simulink model "test_dram_vacc_out"  (Simulink 6.2)
settings: Solver=ode45  StartTime=0.0  StopTime=30000  RelTol=1e-3
undefined symbols (not defined in the file): ant_bits, blockCountBits, blockRowBits
libraries: xbsIndex_r3 x678, xps_library x31, casper_library x10
(part 3 of 4)

== system test_dram_vacc_out/dram_vacc1/test_address ==
  address : Inport  Port=1  LatchInput=off
  RWn : Inport  Port=2  LatchInput=off
  cmd_valid : Inport  Port=3  LatchInput=off
  Concat : xbsIndex_r3/Concat  num_inputs=3  explicit_period=on  period=1  dbl_ovrd=off
  Counter : xbsIndex_r3/Counter  cnt_type=Count Limited  n_bits=11  bin_pt=0  arith_type=Unsigned  start_count=0  cnt_to=Inf  cnt_by_val=1  operation=Up  explicit_period=off  period=1  load_pin=off  rst=off  en=on  dbl_ovrd=off  show_param=off  use_rpm=on  gen_core=off
      settings: xl_area=[0, 0, 0, 0, 0, 0, 0]
  Gateway Out1 : xbsIndex_r3/Gateway Out  output_type=Double  nbits=8  bin_pt=6  arith_type=Boolean  quantization=Truncate  overflow=Wrap  hdl_port=off  timing_constraint=None  locs_specified=off  LOCs={}  needs_fixed_name=off  show_param=off
      settings: xl_area=[0, 0, 0, 0, 0, 0, 0]
  Gateway Out39 : xbsIndex_r3/Gateway Out  output_type=Double  nbits=8  bin_pt=6  arith_type=Boolean  quantization=Truncate  overflow=Wrap  hdl_port=off  timing_constraint=None  locs_specified=off  LOCs={}  needs_fixed_name=off  show_param=off
      settings: xl_area=[0, 0, 0, 0, 0, 0, 0]
  Gateway Out43 : xbsIndex_r3/Gateway Out  output_type=Double  nbits=8  bin_pt=6  arith_type=Boolean  quantization=Truncate  overflow=Wrap  hdl_port=off  timing_constraint=None  locs_specified=off  LOCs={}  needs_fixed_name=off  show_param=off
      settings: xl_area=[0, 0, 0, 0, 0, 0, 0]
  Inverter2 : xbsIndex_r3/Inverter  latency=0  explicit_period=off  period=1  en=off  dbl_ovrd=off  show_param=off
      settings: xl_area=[0, 0, 0, 0, 0, 0, 0]
  Logical2 : xbsIndex_r3/Logical  logical_function=AND  inputs=2  precision=Full  arith_type=Unsigned  n_bits=8  bin_pt=2  align_bp=on  latency=0  explicit_period=off  period=1  en=off  dbl_ovrd=off  show_param=off
      settings: xl_area=[0, 0, 0, 0, 0, 0, 0]
  Register : xbsIndex_r3/Register  init=0  reg_only_valid=off  explicit_period=off  period=1  rst=off  en=on  out_en=off  dbl_ovrd=off  show_param=off
      settings: xl_area=[0, 0, 0, 0, 0, 0, 0]
  Register1 : xbsIndex_r3/Register  init=0  reg_only_valid=off  explicit_period=off  period=1  rst=off  en=off  out_en=off  dbl_ovrd=off  show_param=off
      settings: xl_area=[0, 0, 0, 0, 0, 0, 0]
  Relational : xbsIndex_r3/Relational  mode=a!=b  latency=1  explicit_period=off  period=1  en=on  dbl_ovrd=off  show_param=off
      settings: xl_area=[0, 0, 0, 0, 0, 0, 0]
  Scope2 : Scope  NumInputPorts=3
      settings: YMin=8.55~0.95~-1  YMax=9.45~1.05~1  SaveName=ScopeData10
  Slice1 : xbsIndex_r3/Slice  mode=Lower Bit Location + Width  nbits=2  bit1=0  base1=MSB of Input  bit0=28  base0=LSB of Input  boolean_output=off  explicit_period=off  period=1  dbl_ovrd=off
  Slice2 : xbsIndex_r3/Slice  mode=Lower Bit Location + Width  nbits=8  bit1=0  base1=MSB of Input  bit0=20  base0=LSB of Input  boolean_output=off  explicit_period=off  period=1  dbl_ovrd=off
  Slice3 : xbsIndex_r3/Slice  mode=Lower Bit Location + Width  nbits=1  bit1=0  base1=MSB of Input  bit0=13  base0=LSB of Input  boolean_output=off  explicit_period=off  period=1  dbl_ovrd=off
  bram : xps_library/Shared BRAM  Tag=xps:bram  arith_type="Signed  (2's comp)"  addr_width=11  data_width=32  data_bin_pt=0  init_vals=[1:2^11]  sample_rate=1
  posedge : casper_library/Misc/posedge  Tag=Rising Edge Detector
  wires:
  address/1 -> Slice1/1, Slice2/1, Slice3/1
  Slice3/1 -> Concat/1
  Slice2/1 -> Concat/2
  Slice1/1 -> Concat/3
  RWn/1 -> Inverter2/1
  cmd_valid/1 -> Logical2/2
  Inverter2/1 -> Logical2/1
  Concat/1 -> Register/1, Relational/2
  Logical2/1 -> Register/2, Relational/3
  Register/1 -> Relational/1, Register1/1
  Relational/1 -> posedge/1
  Counter/1 -> bram/1, Gateway Out39/1
  Register1/1 -> bram/2, Gateway Out43/1
  Gateway Out39/1 -> Scope2/1
  Gateway Out43/1 -> Scope2/2
  posedge/1 -> Counter/1, bram/3, Gateway Out1/1
  Gateway Out1/1 -> Scope2/3

== system test_dram_vacc_out/dram_vacc1/test_index ==
  address : Inport  Port=1  LatchInput=off
  RWn : Inport  Port=2  LatchInput=off
  cmd_valid : Inport  Port=3  LatchInput=off
  data : Inport  Port=4  LatchInput=off
  Concat1 : xbsIndex_r3/Concat  num_inputs=2  explicit_period=on  period=1  dbl_ovrd=off
  Convert : xbsIndex_r3/Convert  Orientation=up  arith_type=Boolean  n_bits=8  bin_pt=6  quantization=Truncate  overflow=Wrap  latency=0  explicit_period=on  period=1  dbl_ovrd=off  show_param=off  inserted_by_tool=off  pipeline=off
      settings: xl_area=[0, 0, 0, 0, 0, 0, 0]
  Convert1 : xbsIndex_r3/Convert  arith_type=Unsigned  n_bits=32  bin_pt=0  quantization=Truncate  overflow=Wrap  latency=0  explicit_period=on  period=1  dbl_ovrd=off  show_param=off  inserted_by_tool=off  pipeline=off
      settings: xl_area=[0, 0, 0, 0, 0, 0, 0]
  Counter : xbsIndex_r3/Counter  cnt_type=Count Limited  n_bits=13  bin_pt=0  arith_type=Unsigned  start_count=0  cnt_to=Inf  cnt_by_val=1  operation=Up  explicit_period=off  period=1  load_pin=off  rst=off  en=on  dbl_ovrd=off  show_param=off  use_rpm=on  gen_core=off
      settings: xl_area=[0, 0, 0, 0, 0, 0, 0]
  Gateway Out{1..3,39,43} (5 alike) : xbsIndex_r3/Gateway Out  output_type=Double  nbits=8  bin_pt=6  arith_type=Boolean  quantization=Truncate  overflow=Wrap  hdl_port=off  timing_constraint=None  locs_specified=off  LOCs={}  needs_fixed_name=off  show_param=off
      settings: xl_area=[0, 0, 0, 0, 0, 0, 0]
  Inverter2 : xbsIndex_r3/Inverter  latency=0  explicit_period=off  period=1  en=off  dbl_ovrd=off  show_param=off
      settings: xl_area=[0, 0, 0, 0, 0, 0, 0]
  Logical2 : xbsIndex_r3/Logical  logical_function=AND  inputs=2  precision=Full  arith_type=Unsigned  n_bits=8  bin_pt=2  align_bp=on  latency=0  explicit_period=off  period=1  en=off  dbl_ovrd=off  show_param=off
      settings: xl_area=[0, 0, 0, 0, 0, 0, 0]
  Register : xbsIndex_r3/Register  init=0  reg_only_valid=off  explicit_period=off  period=1  rst=off  en=off  out_en=off  dbl_ovrd=off  show_param=off
      settings: xl_area=[0, 0, 0, 0, 0, 0, 0]
  Relational1 : xbsIndex_r3/Relational  mode=a=b  latency=1  explicit_period=off  period=1  en=on  dbl_ovrd=off  show_param=off
      settings: xl_area=[0, 0, 0, 0, 0, 0, 0]
  Scope2 : Scope  NumInputPorts=5
      settings: YMin=13~0~0~0~0  YMax=16~1000~1~400~1  SaveName=ScopeData10
  Slice1 : xbsIndex_r3/Slice  mode=Lower Bit Location + Width  nbits=14  bit1=0  base1=MSB of Input  bit0=0  base0=LSB of Input  boolean_output=off  explicit_period=off  period=1  dbl_ovrd=off
  Slice4 : xbsIndex_r3/Slice  mode=Lower Bit Location + Width  nbits=32  bit1=0  base1=MSB of Input  bit0=0  base0=LSB of Input  boolean_output=off  explicit_period=off  period=1  dbl_ovrd=off
  bram : xps_library/Shared BRAM  Tag=xps:bram  arith_type=Unsigned  addr_width=13  data_width=32  data_bin_pt=0  init_vals=[1:2^11]  sample_rate=1
  clm_slice : xbsIndex_r3/Slice  mode=Lower Bit Location + Width  nbits=8  bit1=0  base1=MSB of Input  bit0=5  base0=LSB of Input  boolean_output=off  explicit_period=off  period=1  dbl_ovrd=off
  cnt : xps_library/software register  Tag=xps:sw_reg  io_dir=To Processor  arith_type=Unsigned  bitwidth=32  bin_pt=0  sample_period=1  gw_name=test_dram_vacc_out_dram_vacc1_test_index_cnt_user_data_in
  master_reset_sim1 : Constant  Value=4
  posedge2 : casper_library/Misc/posedge  Tag=Rising Edge Detector
  position : xps_library/software register  Tag=xps:sw_reg  io_dir=From Processor  arith_type=Unsigned  bitwidth=32  bin_pt=0  sample_period=1  gw_name=test_dram_vacc_out_dram_vacc1_test_index_position_user_data_out
  row_slice : xbsIndex_r3/Slice  mode=Lower Bit Location + Width  nbits=6  bit1=0  base1=MSB of Input  bit0=14  base0=LSB of Input  boolean_output=off  explicit_period=off  period=1  dbl_ovrd=off
  wires:
  Gateway Out43/1 -> Scope2/2
  Gateway Out39/1 -> Scope2/1
  Counter/1 -> bram/1, Gateway Out39/1, Convert1/1
  Inverter2/1 -> Logical2/1
  cmd_valid/1 -> Logical2/2
  RWn/1 -> Inverter2/1
  address/1 -> clm_slice/1, row_slice/1
  master_reset_sim1/1 -> position/1
  data/1 -> Slice4/1
  row_slice/1 -> Concat1/1
  clm_slice/1 -> Concat1/2
  position/1 -> Slice1/1
  Concat1/1 -> Relational1/2, Gateway Out2/1
  Logical2/1 -> Convert/1, Gateway Out3/1
  Relational1/1 -> posedge2/1
  posedge2/1 -> Counter/1, bram/3, Gateway Out1/1
  Slice4/1 -> Register/1
  Gateway Out1/1 -> Scope2/3
  Register/1 -> bram/2, Gateway Out43/1
  Slice1/1 -> Relational1/1
  Convert/1 -> Relational1/3
  Convert1/1 -> cnt/1
  Gateway Out2/1 -> Scope2/4
  Gateway Out3/1 -> Scope2/5

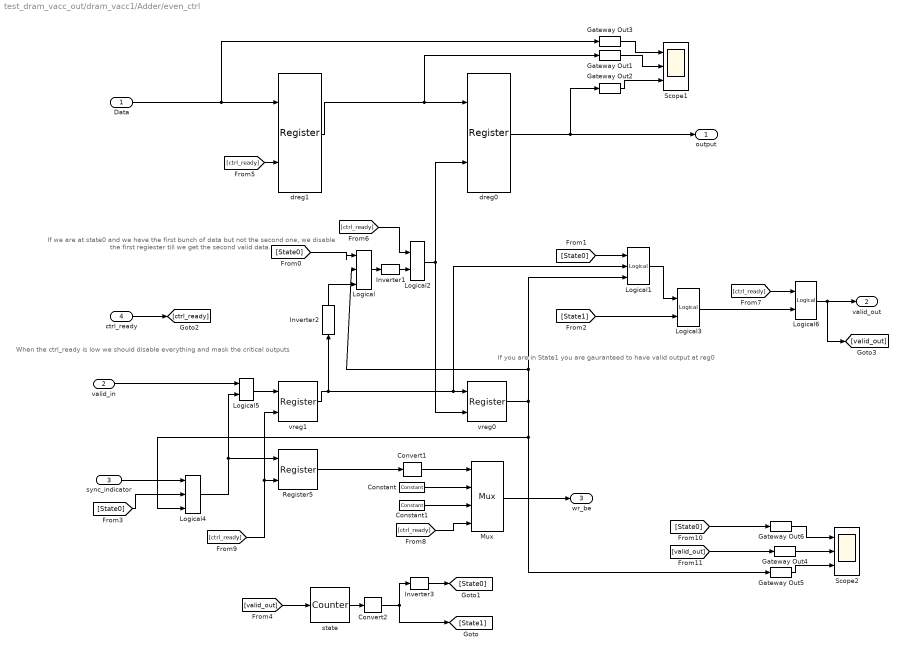
== system test_dram_vacc_out/dram_vacc1/Adder/even_ctrl ==
  note: If we are at state0
      | and we have the first bunch of data
      | but not the second one,
      | we disable the first regiester till we
      | get the second valid  data.
  note: When the ctrl_ready is low
      | we should disable everything
      | and mask the critical outputs
  note: If you are in State1
      | you are gauranteed to have
      | valid output at reg0
  Data : Inport  Port=1  LatchInput=off
  valid_in : Inport  Port=2  LatchInput=off
  sync_indicator : Inport  Port=3  LatchInput=off
  ctrl_ready : Inport  Port=4  LatchInput=off
  Constant : xbsIndex_r3/Constant  const=2^18-1  equ=P=C  arith_type=Unsigned  n_bits=18  bin_pt=0  opselect=C  inp2=PCIN>>17  opr=+  inp1=P  carry=CIN  iostate=0  explicit_period=on  period=1  dbl_ovrd=off
  Constant1 : xbsIndex_r3/Constant  const=0  equ=P=C  arith_type=Unsigned  n_bits=18  bin_pt=0  opselect=C  inp2=PCIN>>17  opr=+  inp1=P  carry=CIN  iostate=0  explicit_period=on  period=1  dbl_ovrd=off
  Convert1 : xbsIndex_r3/Convert  arith_type=Boolean  n_bits=1  bin_pt=0  quantization=Truncate  overflow=Wrap  latency=0  explicit_period=off  period=1  dbl_ovrd=off  show_param=off  inserted_by_tool=off  pipeline=off
      settings: xl_area=[0, 0, 0, 0, 0, 0, 0]
  Convert2 : xbsIndex_r3/Convert  arith_type=Boolean  n_bits=1  bin_pt=0  quantization=Truncate  overflow=Wrap  latency=0  explicit_period=off  period=1  dbl_ovrd=off  show_param=off  inserted_by_tool=off  pipeline=off
      settings: xl_area=[0, 0, 0, 0, 0, 0, 0]
  Gateway Out{1..6} (6 alike) : xbsIndex_r3/Gateway Out  output_type=Double  nbits=8  bin_pt=6  arith_type=Boolean  quantization=Truncate  overflow=Wrap  hdl_port=off  timing_constraint=None  locs_specified=off  LOCs={}  needs_fixed_name=off  show_param=off
      settings: xl_area=[0, 0, 0, 0, 0, 0, 0]
  Inverter1 : xbsIndex_r3/Inverter  latency=0  explicit_period=off  period=1  en=off  dbl_ovrd=off  show_param=off
      settings: xl_area=[0, 0, 0, 0, 0, 0, 0]
  Inverter2 : xbsIndex_r3/Inverter  Orientation=up  latency=0  explicit_period=off  period=1  en=off  dbl_ovrd=off  show_param=off
      settings: xl_area=[0, 0, 0, 0, 0, 0, 0]
  Inverter3 : xbsIndex_r3/Inverter  latency=0  explicit_period=off  period=1  en=off  dbl_ovrd=off  show_param=off
      settings: xl_area=[0, 0, 0, 0, 0, 0, 0]
  Logical : xbsIndex_r3/Logical  logical_function=AND  inputs=3  precision=Full  arith_type=Unsigned  n_bits=8  bin_pt=2  align_bp=on  latency=0  explicit_period=off  period=1  en=off  dbl_ovrd=off  show_param=off
      settings: xl_area=[0, 0, 0, 0, 0, 0, 0]
  Logical1 : xbsIndex_r3/Logical  logical_function=AND  inputs=3  precision=Full  arith_type=Unsigned  n_bits=8  bin_pt=2  align_bp=on  latency=0  explicit_period=off  period=1  en=off  dbl_ovrd=off  show_param=off
      settings: xl_area=[0, 0, 0, 0, 0, 0, 0]
  Logical2 : xbsIndex_r3/Logical  logical_function=AND  inputs=2  precision=Full  arith_type=Unsigned  n_bits=8  bin_pt=2  align_bp=on  latency=0  explicit_period=off  period=1  en=off  dbl_ovrd=off  show_param=off
      settings: xl_area=[0, 0, 0, 0, 0, 0, 0]
  Logical3 : xbsIndex_r3/Logical  logical_function=OR  inputs=2  precision=Full  arith_type=Unsigned  n_bits=8  bin_pt=2  align_bp=on  latency=0  explicit_period=off  period=1  en=off  dbl_ovrd=off  show_param=off
      settings: xl_area=[0, 0, 0, 0, 0, 0, 0]
  Logical4 : xbsIndex_r3/Logical  logical_function=AND  inputs=3  precision=Full  arith_type=Unsigned  n_bits=8  bin_pt=2  align_bp=on  latency=0  explicit_period=off  period=1  en=off  dbl_ovrd=off  show_param=off
      settings: xl_area=[0, 0, 0, 0, 0, 0, 0]
  Logical5 : xbsIndex_r3/Logical  logical_function=OR  inputs=2  precision=Full  arith_type=Unsigned  n_bits=8  bin_pt=2  align_bp=on  latency=0  explicit_period=off  period=1  en=off  dbl_ovrd=off  show_param=off
      settings: xl_area=[0, 0, 0, 0, 0, 0, 0]
  Logical6 : xbsIndex_r3/Logical  logical_function=AND  inputs=2  precision=Full  arith_type=Unsigned  n_bits=8  bin_pt=2  align_bp=on  latency=0  explicit_period=off  period=1  en=off  dbl_ovrd=off  show_param=off
      settings: xl_area=[0, 0, 0, 0, 0, 0, 0]
  Mux : xbsIndex_r3/Mux  inputs=2  precision=Full  arith_type="Signed  (2's comp)"  n_bits=8  bin_pt=2  quantization=Truncate  overflow=Wrap  latency=1  explicit_period=off  period=1  en=on  dbl_ovrd=off  show_param=off  mux_type=off  use_rpm=off  gen_core=off
      settings: xl_area=[0, 0, 0, 0, 0, 0, 0]
  Register5 : xbsIndex_r3/Register  init=0  reg_only_valid=off  explicit_period=off  period=1  rst=off  en=on  out_en=off  dbl_ovrd=off  show_param=off
      settings: xl_area=[0, 0, 0, 0, 0, 0, 0]
  Scope1 : Scope  NumInputPorts=3
      settings: YMin=0~0~0  YMax=1100~1~1  SaveName=ScopeData2
  Scope2 : Scope  NumInputPorts=3
      settings: YMin=0~0~0  YMax=1100~1~1
  dreg0 : xbsIndex_r3/Register  init=0  reg_only_valid=off  explicit_period=on  period=1  rst=off  en=on  out_en=off  dbl_ovrd=off  show_param=off
      settings: xl_area=[0, 0, 0, 0, 0, 0, 0]
  dreg1 : xbsIndex_r3/Register  init=0  reg_only_valid=off  explicit_period=off  period=1  rst=off  en=on  out_en=off  dbl_ovrd=off  show_param=off
      settings: xl_area=[0, 0, 0, 0, 0, 0, 0]
  state : xbsIndex_r3/Counter  cnt_type=Free Running  n_bits=1  bin_pt=0  arith_type=Unsigned  start_count=0  cnt_to=Inf  cnt_by_val=1  operation=Up  explicit_period=on  period=1  load_pin=off  rst=off  en=on  dbl_ovrd=off  show_param=off  use_rpm=on  gen_core=off
      settings: xl_area=[0, 0, 0, 0, 0, 0, 0]
  vreg0 : xbsIndex_r3/Register  init=0  reg_only_valid=off  explicit_period=on  period=1  rst=off  en=on  out_en=off  dbl_ovrd=off  show_param=off
      settings: xl_area=[0, 0, 0, 0, 0, 0, 0]
  vreg1 : xbsIndex_r3/Register  init=0  reg_only_valid=off  explicit_period=on  period=1  rst=off  en=on  out_en=off  dbl_ovrd=off  show_param=off
      settings: xl_area=[0, 0, 0, 0, 0, 0, 0]
  output : Outport
  valid_out : Outport  Port=2
  wr_be : Outport  Port=3
  wires:
  Data/1 -> dreg1/1, Gateway Out3/1
  valid_in/1 -> Logical5/1
  vreg1/1 -> vreg0/1, Logical1/2, Inverter2/1
  dreg1/1 -> dreg0/1, Gateway Out1/1
  dreg0/1 -> output/1, Gateway Out2/1
  state/1 -> Convert2/1
  [State0] -> Logical/1
  vreg0/1 -> Logical/2, Logical1/3, Logical4/3, Gateway Out5/1
  Logical/1 -> Inverter1/1
  [State0] -> Logical1/1
  Inverter3/1 -> [State0]
  [State1] -> Logical3/2
  Logical1/1 -> Logical3/1
  ctrl_ready/1 -> [ctrl_ready]
  Logical3/1 -> Logical6/2
  Inverter2/1 -> Logical/3
  [valid_out] -> state/1
  sync_indicator/1 -> Logical4/1
  [State0] -> Logical4/2
  Mux/1 -> wr_be/1
  Logical5/1 -> vreg1/1
  Logical4/1 -> Logical5/2, Register5/1
  Register5/1 -> Convert1/1
  Constant/1 -> Mux/2
  Constant1/1 -> Mux/3
  [ctrl_ready] -> dreg1/2
  Logical6/1 -> valid_out/1, [valid_out]
  [ctrl_ready] -> Logical6/1
  [ctrl_ready] -> Mux/4
  [ctrl_ready] -> vreg1/2, Register5/2
  Gateway Out6/1 -> Scope2/1
  Gateway Out4/1 -> Scope2/2
  Gateway Out5/1 -> Scope2/3
  [State0] -> Gateway Out6/1
  [valid_out] -> Gateway Out4/1
  Gateway Out3/1 -> Scope1/1
  Gateway Out1/1 -> Scope1/2
  Gateway Out2/1 -> Scope1/3
  Convert1/1 -> Mux/1
  Convert2/1 -> [State1], Inverter3/1
  Inverter1/1 -> Logical2/2
  [ctrl_ready] -> Logical2/1
  Logical2/1 -> dreg0/2, vreg0/2

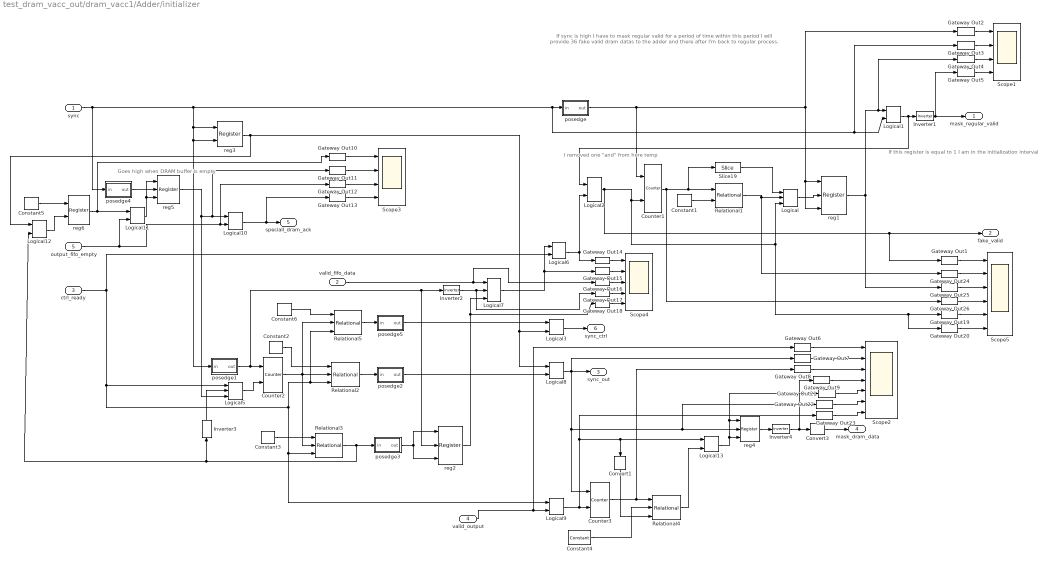
== system test_dram_vacc_out/dram_vacc1/Adder/initializer ==
  note: I removed one "and"
      | from here temp
  note: If this register is equal to 1 I am
      | in the initialization interval
  note: If sync is high I have to mask regular valid for a period of time
      | within this period I will provide 36 fake valid dram datas to the adder and there after I'm back to
      | regular process.
  note: Goes high when DRAM
      | buffer is empty
  sync : Inport  Port=1  LatchInput=off
  valid_fifo_data : Inport  Port=2  LatchInput=off
  ctrl_ready : Inport  Port=3  LatchInput=off
  valid_output : Inport  Port=4  LatchInput=off
  output_fifo_empty : Inport  Port=5  LatchInput=off
  Constant1 : xbsIndex_r3/Constant  const=34  equ=P=C  arith_type=Unsigned  n_bits=6  bin_pt=0  opselect=C  inp2=PCIN>>17  opr=+  inp1=P  carry=CIN  iostate=0  explicit_period=on  period=1  dbl_ovrd=off
  Constant2 : xbsIndex_r3/Constant  const=7  equ=P=C  arith_type=Unsigned  n_bits=4  bin_pt=0  opselect=C  inp2=PCIN>>17  opr=+  inp1=P  carry=CIN  iostate=0  explicit_period=on  period=1  dbl_ovrd=off
  Constant3 : xbsIndex_r3/Constant  const=14  equ=P=C  arith_type=Unsigned  n_bits=4  bin_pt=0  opselect=C  inp2=PCIN>>17  opr=+  inp1=P  carry=CIN  iostate=0  explicit_period=on  period=1  dbl_ovrd=off
  Constant4 : xbsIndex_r3/Constant  const=acc_length-2  equ=P=C  arith_type=Unsigned  n_bits=22  bin_pt=0  opselect=C  inp2=PCIN>>17  opr=+  inp1=P  carry=CIN  iostate=0  explicit_period=on  period=1  dbl_ovrd=off
  Constant5 : xbsIndex_r3/Constant  const=0  equ=P=C  arith_type=Boolean  n_bits=4  bin_pt=0  opselect=C  inp2=PCIN>>17  opr=+  inp1=P  carry=CIN  iostate=0  explicit_period=on  period=1  dbl_ovrd=off
  Constant6 : xbsIndex_r3/Constant  const=4  equ=P=C  arith_type=Unsigned  n_bits=4  bin_pt=0  opselect=C  inp2=PCIN>>17  opr=+  inp1=P  carry=CIN  iostate=0  explicit_period=on  period=1  dbl_ovrd=off
  Convert1 : xbsIndex_r3/Convert  Orientation=down  arith_type=Boolean  n_bits=1  bin_pt=0  quantization=Truncate  overflow=Wrap  latency=0  explicit_period=off  period=1  dbl_ovrd=off  show_param=off  inserted_by_tool=off  pipeline=off
      settings: xl_area=[0, 0, 0, 0, 0, 0, 0]
  Convert3 : xbsIndex_r3/Convert  arith_type=Unsigned  n_bits=1  bin_pt=0  quantization=Truncate  overflow=Wrap  latency=0  explicit_period=off  period=1  dbl_ovrd=off  show_param=off  inserted_by_tool=off  pipeline=off
      settings: xl_area=[0, 0, 0, 0, 0, 0, 0]
  Counter1 : xbsIndex_r3/Counter  cnt_type=Count Limited  n_bits=6  bin_pt=0  arith_type=Unsigned  start_count=0  cnt_to=35  cnt_by_val=1  operation=Up  explicit_period=on  period=1  load_pin=off  rst=on  en=on  dbl_ovrd=off  show_param=off  use_rpm=on  gen_core=off
      settings: xl_area=[0, 0, 0, 0, 0, 0, 0]
  Counter2 : xbsIndex_r3/Counter  cnt_type=Free Running  n_bits=4  bin_pt=0  arith_type=Unsigned  start_count=0  cnt_to=35  cnt_by_val=1  operation=Up  explicit_period=on  period=1  load_pin=off  rst=on  en=on  dbl_ovrd=off  show_param=off  use_rpm=on  gen_core=off
      settings: xl_area=[0, 0, 0, 0, 0, 0, 0]
  Counter3 : xbsIndex_r3/Counter  cnt_type=Free Running  n_bits=22  bin_pt=0  arith_type=Unsigned  start_count=0  cnt_to=35  cnt_by_val=1  operation=Up  explicit_period=on  period=1  load_pin=off  rst=on  en=on  dbl_ovrd=off  show_param=off  use_rpm=on  gen_core=off
      settings: xl_area=[0, 0, 0, 0, 0, 0, 0]
  Gateway Out{1..26} (26 alike) : xbsIndex_r3/Gateway Out  output_type=Double  nbits=8  bin_pt=6  arith_type=Boolean  quantization=Truncate  overflow=Wrap  hdl_port=off  timing_constraint=None  locs_specified=off  LOCs={}  needs_fixed_name=off  show_param=off
      settings: xl_area=[0, 0, 0, 0, 0, 0, 0]
  Inverter1 : xbsIndex_r3/Inverter  latency=0  explicit_period=off  period=1  en=off  dbl_ovrd=off  show_param=off
      settings: xl_area=[0, 0, 0, 0, 0, 0, 0]
  Inverter2 : xbsIndex_r3/Inverter  latency=0  explicit_period=off  period=1  en=off  dbl_ovrd=off  show_param=off
      settings: xl_area=[0, 0, 0, 0, 0, 0, 0]
  Inverter3 : xbsIndex_r3/Inverter  Orientation=up  latency=0  explicit_period=off  period=1  en=off  dbl_ovrd=off  show_param=off
      settings: xl_area=[0, 0, 0, 0, 0, 0, 0]
  Inverter4 : xbsIndex_r3/Inverter  latency=0  explicit_period=off  period=1  en=off  dbl_ovrd=off  show_param=off
      settings: xl_area=[0, 0, 0, 0, 0, 0, 0]
  Logical : xbsIndex_r3/Logical  logical_function=AND  inputs=3  precision=Full  arith_type=Unsigned  n_bits=8  bin_pt=2  align_bp=on  latency=0  explicit_period=on  period=1  en=off  dbl_ovrd=off  show_param=off
      settings: xl_area=[0, 0, 0, 0, 0, 0, 0]
  Logical1 : xbsIndex_r3/Logical  logical_function=OR  inputs=2  precision=Full  arith_type=Unsigned  n_bits=8  bin_pt=2  align_bp=on  latency=0  explicit_period=off  period=1  en=off  dbl_ovrd=off  show_param=off
      settings: xl_area=[0, 0, 0, 0, 0, 0, 0]
  Logical10 : xbsIndex_r3/Logical  logical_function=NOR  inputs=2  precision=Full  arith_type=Unsigned  n_bits=8  bin_pt=2  align_bp=on  latency=0  explicit_period=off  period=1  en=off  dbl_ovrd=off  show_param=off
      settings: xl_area=[0, 0, 0, 0, 0, 0, 0]
  Logical11 : xbsIndex_r3/Logical  logical_function=OR  inputs=2  precision=Full  arith_type=Unsigned  n_bits=8  bin_pt=2  align_bp=on  latency=0  explicit_period=off  period=1  en=off  dbl_ovrd=off  show_param=off
      settings: xl_area=[0, 0, 0, 0, 0, 0, 0]
  Logical{2..3,6,8..9,12..13} (7 alike) : xbsIndex_r3/Logical  logical_function=AND  inputs=2  precision=Full  arith_type=Unsigned  n_bits=8  bin_pt=2  align_bp=on  latency=0  explicit_period=off  period=1  en=off  dbl_ovrd=off  show_param=off
      settings: xl_area=[0, 0, 0, 0, 0, 0, 0]
  Logical5 : xbsIndex_r3/Logical  logical_function=AND  inputs=3  precision=Full  arith_type=Unsigned  n_bits=8  bin_pt=2  align_bp=on  latency=0  explicit_period=off  period=1  en=off  dbl_ovrd=off  show_param=off
      settings: xl_area=[0, 0, 0, 0, 0, 0, 0]
  Logical7 : xbsIndex_r3/Logical  logical_function=AND  inputs=3  precision=Full  arith_type=Unsigned  n_bits=8  bin_pt=2  align_bp=on  latency=0  explicit_period=off  period=1  en=off  dbl_ovrd=off  show_param=off
      settings: xl_area=[0, 0, 0, 0, 0, 0, 0]
  Relational1 : xbsIndex_r3/Relational  mode=a>=b  latency=1  explicit_period=on  period=1  en=off  dbl_ovrd=off  show_param=off
      settings: xl_area=[0, 0, 0, 0, 0, 0, 0]
  Relational2 : xbsIndex_r3/Relational  mode=a<=b  latency=1  explicit_period=on  period=1  en=on  dbl_ovrd=off  show_param=off
      settings: xl_area=[0, 0, 0, 0, 0, 0, 0]
  Relational3 : xbsIndex_r3/Relational  mode=a<=b  latency=1  explicit_period=on  period=1  en=on  dbl_ovrd=off  show_param=off
      settings: xl_area=[0, 0, 0, 0, 0, 0, 0]
  Relational4 : xbsIndex_r3/Relational  mode=a=b  latency=1  explicit_period=on  period=1  en=on  dbl_ovrd=off  show_param=off
      settings: xl_area=[0, 0, 0, 0, 0, 0, 0]
  Relational5 : xbsIndex_r3/Relational  mode=a<=b  latency=1  explicit_period=on  period=1  en=on  dbl_ovrd=off  show_param=off
      settings: xl_area=[0, 0, 0, 0, 0, 0, 0]
  Scope1 : Scope  NumInputPorts=4
      settings: YMin=-1~-1~50~0  YMax=1~1~90~1  SaveName=ScopeData13
  Scope2 : Scope  NumInputPorts=7
      settings: YMin=-1~-1~50~0~-5~-5~-5  YMax=1~1~90~1~5~5~5  SaveName=ScopeData15
  Scope3 : Scope  NumInputPorts=4
      settings: YMin=-1~-1~50~0  YMax=1~1~90~1  SaveName=ScopeData18
  Scope4 : Scope  NumInputPorts=5
      settings: YMin=-1~-1~50~0~-5  YMax=1~1~90~1~5  SaveName=ScopeData31
  Scope5 : Scope  NumInputPorts=6
      settings: YMin=-1~-1~50~0~-5~-5  YMax=1~1~90~1~5~5  SaveName=ScopeData3
  Slice19 : xbsIndex_r3/Slice  mode=Lower Bit Location + Width  nbits=1  bit1=0  base1=MSB of Input  bit0=0  base0=LSB of Input  boolean_output=on  explicit_period=off  period=1  dbl_ovrd=off
  posedge : Subsystem
  posedge1 : Subsystem
  posedge2 : Subsystem
  posedge3 : Subsystem
  posedge4 : Subsystem
  posedge5 : Subsystem
  reg{1..2,4..5} (4 alike) : xbsIndex_r3/Register  init=0  reg_only_valid=off  explicit_period=on  period=1  rst=on  en=on  out_en=off  dbl_ovrd=off  show_param=off
      settings: xl_area=[0, 0, 0, 0, 0, 0, 0]
  reg3 : xbsIndex_r3/Register  init=0  reg_only_valid=off  explicit_period=on  period=1  rst=off  en=on  out_en=off  dbl_ovrd=off  show_param=off
      settings: xl_area=[0, 0, 0, 0, 0, 0, 0]
  reg6 : xbsIndex_r3/Register  init=1  reg_only_valid=off  explicit_period=on  period=1  rst=off  en=on  out_en=off  dbl_ovrd=off  show_param=off
      settings: xl_area=[0, 0, 0, 0, 0, 0, 0]
  mask_regular_valid : Outport
  fake_valid : Outport  Port=2
  sync_out : Outport  Port=3
  mask_dram_data : Outport  Port=4
  speciall_dram_ack : Outport  Port=5
  sync_ctrl : Outport  Port=6
  wires:
  Convert1/1 -> Relational4/3
  Gateway Out23/1 -> Scope2/7
  Gateway Out22/1 -> Scope2/6
  Gateway Out21/1 -> Scope2/5
  Slice19/1 -> Logical/1
  Gateway Out20/1 -> Scope5/6
  Gateway Out19/1 -> Scope5/5
  Gateway Out18/1 -> Scope4/5
  Gateway Out17/1 -> Scope4/4
  Gateway Out16/1 -> Scope4/3
  Gateway Out15/1 -> Scope4/2
  Gateway Out14/1 -> Scope4/1
  Convert3/1 -> mask_dram_data/1
  Relational4/1 -> Logical13/2
  Logical13/1 -> Gateway Out21/1, reg4/1, reg4/3
  reg6/1 -> Gateway Out10/1, Logical11/1
  Logical12/1 -> reg6/2
  Constant5/1 -> reg6/1
  Gateway Out10/1 -> Scope3/1
  Gateway Out13/1 -> Scope3/4
  Gateway Out12/1 -> Scope3/3
  Gateway Out11/1 -> Scope3/2
  Logical11/1 -> reg5/3, reg5/1
  Logical10/1 -> Gateway Out13/1, speciall_dram_ack/1
  output_fifo_empty/1 -> Gateway Out12/1, Logical10/2, Logical11/2
  reg5/1 -> Gateway Out11/1, Logical10/1, Logical5/3
  posedge4/1(out) -> reg5/2
  Gateway Out6/1 -> Scope2/1
  Gateway Out9/1 -> Scope2/4
  Gateway Out8/1 -> Scope2/3
  Gateway Out7/1 -> Scope2/2
  Inverter4/1 -> Convert3/1, Gateway Out9/1
  reg4/1 -> Inverter4/1
  Constant4/1 -> Relational4/2
  Counter3/1 -> Gateway Out8/1, Relational4/1
  valid_output/1 -> Gateway Out6/1, Logical9/2
  Logical9/1 -> Convert1/1, Logical13/1, Gateway Out23/1, Counter3/2
  reg3/1 -> Logical12/1, Logical8/1, Logical3/2
  posedge2/1(out) -> Logical8/2
  Logical8/1 -> Gateway Out7/1, Gateway Out22/1, reg4/2, Counter3/1, sync_out/1
  Inverter3/1 -> Logical5/2
  Logical5/1 -> Counter2/2
  Logical7/1 -> Gateway Out15/1, Logical6/1
  valid_fifo_data/1 -> Gateway Out16/1, Logical7/1
  Inverter2/1 -> Gateway Out17/1, Logical7/2
  reg2/1 -> Gateway Out18/1, Logical7/3
  posedge3/1(out) -> reg2/3, reg2/1
  Relational3/1 -> Logical12/2, Inverter3/1, posedge3/1(in)
  Constant3/1 -> Relational3/1
  Relational2/1 -> posedge2/1(in)
  Constant2/1 -> Relational2/1
  Counter2/1 -> Relational3/2, Relational2/2, Relational5/2
  posedge1/1(out) -> Inverter2/1, reg2/2, Counter2/1
  Inverter1/1 -> Gateway Out5/1, mask_regular_valid/1
  Logical/1 -> reg1/2
  Logical6/1 -> Gateway Out14/1, Logical2/2
  ctrl_ready/1 -> Logical9/1, Relational3/3, Relational2/3, Relational5/3, Logical5/1, Logical6/2
  Relational1/1 -> Logical/2, Gateway Out24/1
  reg1/1 -> Gateway Out25/1, Gateway Out4/1, Logical1/1
  Constant1/1 -> Relational1/2
  Counter1/1 -> Slice19/1, Relational1/1, Gateway Out26/1
  Logical2/1 -> Counter1/2, Gateway Out20/1, Gateway Out19/1, Logical/3, Gateway Out1/1, fake_valid/1
  Logical1/1 -> Logical2/1, Inverter1/1
  posedge/1(out) -> Counter1/1, reg1/3, reg1/1, Gateway Out2/1
  sync/1 -> posedge4/1(in), reg3/1, reg3/2, posedge1/1(in), Gateway Out3/1, Logical1/2, posedge/1(in)
  Gateway Out2/1 -> Scope1/1
  Gateway Out5/1 -> Scope1/4
  Gateway Out4/1 -> Scope1/3
  Gateway Out3/1 -> Scope1/2
  Gateway Out1/1 -> Scope5/1
  Gateway Out26/1 -> Scope5/4
  Gateway Out25/1 -> Scope5/3
  Gateway Out24/1 -> Scope5/2
  Constant6/1 -> Relational5/1
  Relational5/1 -> posedge5/1(in)
  posedge5/1(out) -> Logical3/1
  Logical3/1 -> sync_ctrl/1

== system test_dram_vacc_out/dram_vacc1/RB_reg/Trickle_FWFT ==
  note: We needed a FIFO which brings the valid data automatically to the output.
      | The regular XILINX Fifos are not FWFT (First Word Fall Through).
      | We tried to make one but it was really hard to make one agreeing with the exact specs.
      | This module which we have named it Trickle_FWFT Fifo works very similiarly with minor
      | differences which servers our purpose here in the DRAM VACC module.
  note: The real depth of this module is depth+1.
      | The valid signal will go high with one cycle delay.
  din : Inport  Port=1  LatchInput=off
  we : Inport  Port=2  LatchInput=off
  ack : Inport  Port=3  LatchInput=off
  reset : Inport  Port=4  LatchInput=off
  Convert : xbsIndex_r3/Convert  Orientation=left  arith_type=Boolean  n_bits=8  bin_pt=6  quantization=Truncate  overflow=Wrap  latency=0  explicit_period=on  period=1  dbl_ovrd=off  show_param=off  inserted_by_tool=off  pipeline=off
      settings: xl_area=[0, 0, 0, 0, 0, 0, 0]
  Convert3 : xbsIndex_r3/Convert  arith_type=Boolean  n_bits=8  bin_pt=6  quantization=Truncate  overflow=Wrap  latency=0  explicit_period=off  period=1  dbl_ovrd=off  show_param=off  inserted_by_tool=off  pipeline=off
      settings: xl_area=[0, 0, 0, 0, 0, 0, 0]
  FIFO : xbsIndex_r3/FIFO  depth=16  percent_nbits=1  store_only_valid=on  init_zero=on  explicit_period=on  period=1  rst=on  en=off  use_almost_empty=off  almost_empty_offset=6  use_almost_full=off  almost_full_offset=6  dbl_ovrd=off  show_param=off  mem_type=Block RAM  gen_core=off
      settings: xl_area=[0, 0, 0, 0, 0, 0, 0]
  Inverter3 : xbsIndex_r3/Inverter  latency=0  explicit_period=off  period=1  en=off  dbl_ovrd=off  show_param=off
      settings: xl_area=[0, 0, 0, 0, 0, 0, 0]
  Logical2 : xbsIndex_r3/Logical  logical_function=OR  inputs=2  precision=Full  arith_type=Unsigned  n_bits=8  bin_pt=2  align_bp=on  latency=0  explicit_period=on  period=1  en=off  dbl_ovrd=off  show_param=off
      settings: xl_area=[0, 0, 0, 0, 0, 0, 0]
  not_valid : xbsIndex_r3/Register  init=1  reg_only_valid=off  explicit_period=on  period=1  rst=on  en=on  out_en=off  dbl_ovrd=off  show_param=off
      settings: xl_area=[0, 0, 0, 0, 0, 0, 0]
  data_out : Outport
  valid : Outport  Port=2
  full : Outport  Port=3
  %full : Outport  Port=4
  wires:
  din/1 -> FIFO/1
  we/1 -> FIFO/2
  FIFO/2 -> not_valid/1
  ack/1 -> Logical2/2
  FIFO/1 -> data_out/1
  FIFO/4 -> full/1
  Inverter3/1 -> Convert3/1
  reset/1 -> FIFO/4, not_valid/2
  Logical2/1 -> FIFO/3, not_valid/3
  not_valid/1 -> Inverter3/1, Convert/1
  Convert/1 -> Logical2/1
  FIFO/3 -> %full/1
  Convert3/1 -> valid/1

== system test_dram_vacc_out/dram_vacc1/RB_reg/er ==
  dout : Inport  Port=1  LatchInput=off
  valid : Inport  Port=2  LatchInput=off
  Constant : xbsIndex_r3/Constant  const=1  equ=P=C  arith_type=Unsigned  n_bits=128  bin_pt=0  opselect=C  inp2=PCIN>>17  opr=+  inp1=P  carry=CIN  iostate=0  explicit_period=on  period=1  dbl_ovrd=off
  Constant1 : Constant  Value=0
  Delay : xbsIndex_r3/Delay  latency=3  reg_retiming=off  explicit_period=off  period=1  en=off  accept_only_valid=off  init_zero=on  dbl_ovrd=off  show_param=off
      settings: xl_area=[0, 0, 0, 0, 0, 0, 0]
  Logical : xbsIndex_r3/Logical  logical_function=AND  inputs=2  precision=Full  arith_type=Unsigned  n_bits=8  bin_pt=2  align_bp=on  latency=0  explicit_period=off  period=1  en=off  dbl_ovrd=off  show_param=off
      settings: xl_area=[0, 0, 0, 0, 0, 0, 0]
  Register : xbsIndex_r3/Register  init=0  reg_only_valid=off  explicit_period=off  period=1  rst=on  en=on  out_en=off  dbl_ovrd=off  show_param=off
      settings: xl_area=[0, 0, 0, 0, 0, 0, 0]
  Rel : xbsIndex_r3/Relational  mode=a=b  latency=3  explicit_period=off  period=1  en=off  dbl_ovrd=off  show_param=on
      settings: xl_area=[0, 0, 0, 0, 0, 0, 0]
  Slice2 : xbsIndex_r3/Slice  mode=Lower Bit Location + Width  nbits=1  bit1=3  base1=LSB of Input  bit0=0  base0=LSB of Input  boolean_output=on  explicit_period=on  period=1  dbl_ovrd=off
  re : xps_library/software register  Tag=xps:sw_reg  io_dir=From Processor  arith_type=Unsigned  bitwidth=32  bin_pt=0  sample_period=1  gw_name=test_dram_vacc_out_dram_vacc1_RB_reg_er_re_user_data_out
  error : Outport
  wires:
  Constant/1 -> Rel/1
  Rel/1 -> Logical/1
  Delay/1 -> Logical/2
  Logical/1 -> Register/1, Register/3
  re/1 -> Slice2/1
  Constant1/1 -> re/1
  dout/1 -> Rel/2
  valid/1 -> Delay/1
  Register/1 -> error/1
  Slice2/1 -> Register/2

== system test_dram_vacc_out/dram_vacc1/RB_reg/posedge ==
  in : Inport  Port=1  LatchInput=off
  Delay : xbsIndex_r3/Delay  latency=1  reg_retiming=off  explicit_period=off  period=1  en=off  accept_only_valid=off  init_zero=on  dbl_ovrd=off  show_param=off
      settings: xl_area=[0, 0, 0, 0, 0, 0, 0]
  Inverter2 : xbsIndex_r3/Inverter  latency=0  explicit_period=off  period=1  en=off  dbl_ovrd=off  show_param=off
      settings: xl_area=[0, 0, 0, 0, 0, 0, 0]
  Logical : xbsIndex_r3/Logical  logical_function=AND  inputs=2  precision=Full  arith_type=Unsigned  n_bits=8  bin_pt=2  align_bp=on  latency=0  explicit_period=off  period=1  en=off  dbl_ovrd=off  show_param=off
      settings: xl_area=[0, 0, 0, 0, 0, 0, 0]
  out : Outport
  wires:
  Inverter2/1 -> Logical/1
  Logical/1 -> out/1
  in/1 -> Logical/2, Delay/1
  Delay/1 -> Inverter2/1

== system test_dram_vacc_out/dram_vacc1/ctrl_unit/RB_active_or_finish ==
  enable_rb_addr : Inport  Orientation=down  Port=1  LatchInput=off
  sync : Inport  Port=2  LatchInput=off
  Constant3 : xbsIndex_r3/Constant  const=acc_length/2  equ=P=C  arith_type=Unsigned  n_bits=32  bin_pt=0  opselect=C  inp2=PCIN>>17  opr=+  inp1=P  carry=CIN  iostate=0  explicit_period=on  period=1  dbl_ovrd=off
  Counter1 : xbsIndex_r3/Counter  cnt_type=Free Running  n_bits=32  bin_pt=0  arith_type=Unsigned  start_count=0  cnt_to=2*burst_length-1  cnt_by_val=1  operation=Up  explicit_period=on  period=1  load_pin=off  rst=on  en=on  dbl_ovrd=off  show_param=off  use_rpm=on  gen_core=off
      settings: xl_area=[0, 0, 0, 0, 0, 0, 0]
  Inverter6 : xbsIndex_r3/Inverter  latency=0  explicit_period=off  period=1  en=off  dbl_ovrd=off  show_param=off
      settings: xl_area=[0, 0, 0, 0, 0, 0, 0]
  Inverter9 : xbsIndex_r3/Inverter  latency=0  explicit_period=off  period=1  en=off  dbl_ovrd=off  show_param=off
      settings: xl_area=[0, 0, 0, 0, 0, 0, 0]
  Logical13 : xbsIndex_r3/Logical  logical_function=AND  inputs=3  precision=Full  arith_type=Unsigned  n_bits=8  bin_pt=2  align_bp=on  latency=0  explicit_period=on  period=1  en=off  dbl_ovrd=off  show_param=off
      settings: xl_area=[0, 0, 0, 0, 0, 0, 0]
  Logical14 : xbsIndex_r3/Logical  logical_function=AND  inputs=2  precision=Full  arith_type=Unsigned  n_bits=8  bin_pt=2  align_bp=on  latency=0  explicit_period=on  period=1  en=off  dbl_ovrd=off  show_param=off
      settings: xl_area=[0, 0, 0, 0, 0, 0, 0]
  Logical7 : xbsIndex_r3/Logical  logical_function=AND  inputs=2  precision=Full  arith_type=Unsigned  n_bits=8  bin_pt=2  align_bp=on  latency=0  explicit_period=on  period=1  en=off  dbl_ovrd=off  show_param=off
      settings: xl_area=[0, 0, 0, 0, 0, 0, 0]
  Relational3 : xbsIndex_r3/Relational  mode=a=b  latency=1  explicit_period=on  period=1  en=off  dbl_ovrd=off  show_param=off
      settings: xl_area=[0, 0, 0, 0, 0, 0, 0]
  system_start : xbsIndex_r3/Register  init=0  reg_only_valid=off  explicit_period=off  period=1  rst=off  en=on  out_en=off  dbl_ovrd=off  show_param=off
      settings: xl_area=[0, 0, 0, 0, 0, 0, 0]
  system_start1 : xbsIndex_r3/Register  init=0  reg_only_valid=off  explicit_period=off  period=1  rst=off  en=on  out_en=off  dbl_ovrd=off  show_param=off
      settings: xl_area=[0, 0, 0, 0, 0, 0, 0]
  system_start2 : xbsIndex_r3/Register  init=0  reg_only_valid=off  explicit_period=off  period=1  rst=on  en=on  out_en=off  dbl_ovrd=off  show_param=off
      settings: xl_area=[0, 0, 0, 0, 0, 0, 0]
  rb_active : Outport
  wires:
  Logical13/1 -> rb_active/1
  sync/1 -> system_start2/2, Counter1/1, system_start/2, system_start/1, Logical14/1, Inverter9/1
  enable_rb_addr/1 -> Logical7/1, Counter1/2
  Inverter9/1 -> Logical13/3
  system_start1/1 -> Logical13/2
  Logical14/1 -> system_start1/2, system_start1/1
  Inverter6/1 -> Logical13/1
  Relational3/1 -> Logical7/2
  Logical7/1 -> system_start2/3, system_start2/1
  Constant3/1 -> Relational3/2
  Counter1/1 -> Relational3/1
  system_start2/1 -> Inverter6/1
  system_start/1 -> Logical14/2

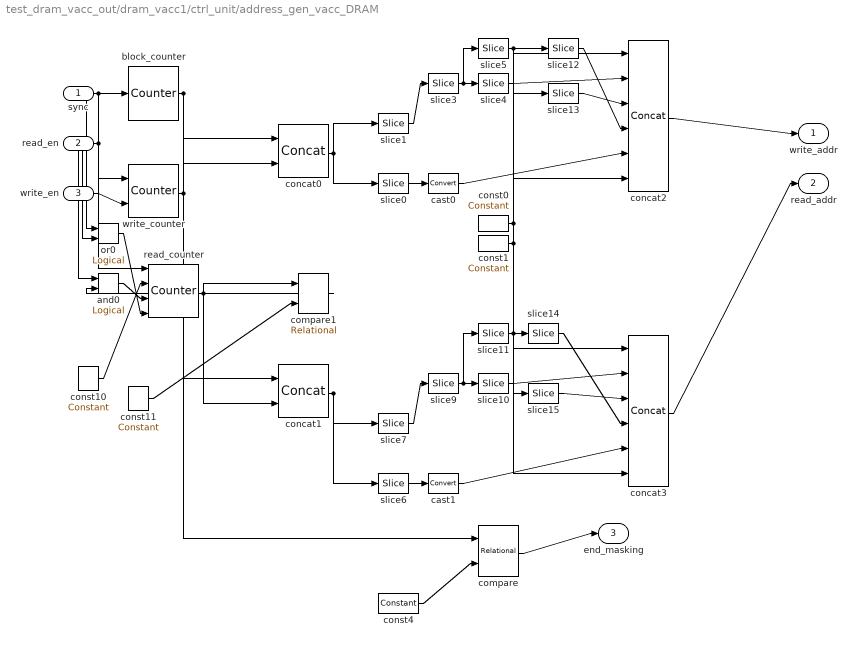
== system test_dram_vacc_out/dram_vacc1/ctrl_unit/address_gen_vacc_DRAM ==
  sync : Inport  Port=1  LatchInput=off
  read_en : Inport  Port=2  LatchInput=off
  write_en : Inport  Port=3  LatchInput=off
  and0 : xbsIndex_r3/Logical  logical_function=AND  inputs=2  precision=Full  arith_type=Unsigned  n_bits=8  bin_pt=2  align_bp=on  latency=0  explicit_period=off  period=1  en=off  dbl_ovrd=off  show_param=off
      settings: xl_area=[0, 0, 0, 0, 0, 0, 0]
  block_counter : xbsIndex_r3/Counter  cnt_type=Free Running  n_bits=blockCountBits  bin_pt=0  arith_type=Unsigned  start_count=2^blockCountBits-1  cnt_to=Inf  cnt_by_val=1  operation=Up  explicit_period=off  period=1  load_pin=off  rst=off  en=on  dbl_ovrd=off  show_param=off  use_rpm=on  gen_core=off
      settings: xl_area=[0, 0, 0, 0, 0, 0, 0]
  cast0 : xbsIndex_r3/Convert  arith_type=Unsigned  n_bits=8  bin_pt=0  quantization=Truncate  overflow=Wrap  latency=0  explicit_period=off  period=1  dbl_ovrd=off  show_param=off  inserted_by_tool=off  pipeline=off
      settings: xl_area=[0, 0, 0, 0, 0, 0, 0]
  cast1 : xbsIndex_r3/Convert  arith_type=Unsigned  n_bits=8  bin_pt=0  quantization=Truncate  overflow=Wrap  latency=0  explicit_period=off  period=1  dbl_ovrd=off  show_param=off  inserted_by_tool=off  pipeline=off
      settings: xl_area=[0, 0, 0, 0, 0, 0, 0]
  compare : xbsIndex_r3/Relational  mode=a=b  latency=1  explicit_period=off  period=1  en=off  dbl_ovrd=off  show_param=off
      settings: xl_area=[0, 0, 0, 0, 0, 0, 0]
  compare1 : xbsIndex_r3/Relational  mode=a=b  latency=1  explicit_period=on  period=1  en=off  dbl_ovrd=off  show_param=off
      settings: xl_area=[0, 0, 0, 0, 0, 0, 0]
  concat0 : xbsIndex_r3/Concat  num_inputs=2  explicit_period=off  period=1  dbl_ovrd=off
  concat1 : xbsIndex_r3/Concat  num_inputs=2  explicit_period=off  period=1  dbl_ovrd=off
  concat2 : xbsIndex_r3/Concat  num_inputs=6  explicit_period=off  period=1  dbl_ovrd=off
  concat3 : xbsIndex_r3/Concat  num_inputs=6  explicit_period=off  period=1  dbl_ovrd=off
  const0 : xbsIndex_r3/Constant  const=0  equ=P=C  arith_type=Unsigned  n_bits=5  bin_pt=0  opselect=C  inp2=PCIN>>17  opr=+  inp1=P  carry=CIN  iostate=0  explicit_period=off  period=1  dbl_ovrd=off
  const1 : xbsIndex_r3/Constant  const=0  equ=P=C  arith_type=Unsigned  n_bits=2  bin_pt=0  opselect=C  inp2=PCIN>>17  opr=+  inp1=P  carry=CIN  iostate=0  explicit_period=off  period=1  dbl_ovrd=off
  const10 : xbsIndex_r3/Constant  const=valid_length/2  equ=P=C  arith_type=Unsigned  n_bits=counterBitWidth  bin_pt=0  opselect=C  inp2=PCIN>>17  opr=+  inp1=P  carry=CIN  iostate=0  explicit_period=on  period=1  dbl_ovrd=off
  const11 : xbsIndex_r3/Constant  const=acc_length/2-1  equ=P=C  arith_type=Unsigned  n_bits=counterBitWidth  bin_pt=0  opselect=C  inp2=PCIN>>17  opr=+  inp1=P  carry=CIN  iostate=0  explicit_period=on  period=1  dbl_ovrd=off
  const4 : xbsIndex_r3/Constant  const=acc_length/2-1  equ=P=C  arith_type=Unsigned  n_bits=counterBitWidth  bin_pt=0  opselect=C  inp2=PCIN>>17  opr=+  inp1=P  carry=CIN  iostate=0  explicit_period=off  period=1  dbl_ovrd=off
  or0 : xbsIndex_r3/Logical  logical_function=OR  inputs=2  precision=Full  arith_type=Unsigned  n_bits=8  bin_pt=2  align_bp=on  latency=0  explicit_period=off  period=1  en=off  dbl_ovrd=off  show_param=off
      settings: xl_area=[0, 0, 0, 0, 0, 0, 0]
  read_counter : xbsIndex_r3/Counter  cnt_type=Free Running  n_bits=counterBitWidth  bin_pt=0  arith_type=Unsigned  start_count=0  cnt_to=Inf  cnt_by_val=1  operation=Up  explicit_period=off  period=1  load_pin=on  rst=on  en=on  dbl_ovrd=off  show_param=off  use_rpm=on  gen_core=off
      settings: xl_area=[0, 0, 0, 0, 0, 0, 0]
  slice0 : xbsIndex_r3/Slice  mode=Lower Bit Location + Width  nbits=colCountBits  bit1=0  base1=MSB of Input  bit0=0  base0=LSB of Input  boolean_output=off  explicit_period=off  period=1  dbl_ovrd=off
  slice1 : xbsIndex_r3/Slice  mode=Upper Bit Location + Width  nbits=blockCountBits+blockRowBits  bit1=0  base1=MSB of Input  bit0=0  base0=LSB of Input  boolean_output=off  explicit_period=off  period=1  dbl_ovrd=off
  slice10 : xbsIndex_r3/Slice  mode=Lower Bit Location + Width  nbits=2  bit1=0  base1=MSB of Input  bit0=0  base0=LSB of Input  boolean_output=off  explicit_period=off  period=1  dbl_ovrd=off
  slice11 : xbsIndex_r3/Slice  mode=Upper Bit Location + Width  nbits=blockCountBits-2  bit1=0  base1=MSB of Input  bit0=0  base0=LSB of Input  boolean_output=off  explicit_period=off  period=1  dbl_ovrd=off
  slice12 : xbsIndex_r3/Slice  mode=Upper Bit Location + Width  nbits=1  bit1=0  base1=MSB of Input  bit0=0  base0=LSB of Input  boolean_output=off  explicit_period=off  period=1  dbl_ovrd=off
  slice13 : xbsIndex_r3/Slice  mode=Lower Bit Location + Width  nbits=blockCountBits-3  bit1=0  base1=MSB of Input  bit0=0  base0=LSB of Input  boolean_output=off  explicit_period=off  period=1  dbl_ovrd=off
  slice14 : xbsIndex_r3/Slice  mode=Upper Bit Location + Width  nbits=1  bit1=0  base1=MSB of Input  bit0=0  base0=LSB of Input  boolean_output=off  explicit_period=off  period=1  dbl_ovrd=off
  slice15 : xbsIndex_r3/Slice  mode=Lower Bit Location + Width  nbits=blockCountBits-3  bit1=0  base1=MSB of Input  bit0=0  base0=LSB of Input  boolean_output=off  explicit_period=off  period=1  dbl_ovrd=off
  slice3 : xbsIndex_r3/Slice  mode=Upper Bit Location + Width  nbits=blockCountBits  bit1=0  base1=MSB of Input  bit0=0  base0=LSB of Input  boolean_output=off  explicit_period=off  period=1  dbl_ovrd=off
  slice4 : xbsIndex_r3/Slice  mode=Lower Bit Location + Width  nbits=2  bit1=0  base1=MSB of Input  bit0=0  base0=LSB of Input  boolean_output=off  explicit_period=off  period=1  dbl_ovrd=off
  slice5 : xbsIndex_r3/Slice  mode=Upper Bit Location + Width  nbits=blockCountBits-2  bit1=0  base1=MSB of Input  bit0=0  base0=LSB of Input  boolean_output=off  explicit_period=off  period=1  dbl_ovrd=off
  slice6 : xbsIndex_r3/Slice  mode=Lower Bit Location + Width  nbits=colCountBits  bit1=0  base1=MSB of Input  bit0=0  base0=LSB of Input  boolean_output=off  explicit_period=off  period=1  dbl_ovrd=off
  slice7 : xbsIndex_r3/Slice  mode=Upper Bit Location + Width  nbits=blockCountBits+blockRowBits  bit1=0  base1=MSB of Input  bit0=0  base0=LSB of Input  boolean_output=off  explicit_period=off  period=1  dbl_ovrd=off
  slice9 : xbsIndex_r3/Slice  mode=Upper Bit Location + Width  nbits=blockCountBits  bit1=0  base1=MSB of Input  bit0=0  base0=LSB of Input  boolean_output=off  explicit_period=off  period=1  dbl_ovrd=off
  write_counter : xbsIndex_r3/Counter  cnt_type=Count Limited  n_bits=counterBitWidth  bin_pt=0  arith_type=Unsigned  start_count=0  cnt_to=acc_length/2-1  cnt_by_val=1  operation=Up  explicit_period=off  period=1  load_pin=off  rst=on  en=on  dbl_ovrd=off  show_param=off  use_rpm=on  gen_core=off
      settings: xl_area=[0, 0, 0, 0, 0, 0, 0]
  write_addr : Outport
  read_addr : Outport  Port=2
  end_masking : Outport  Port=3
  wires:
  const1/1 -> concat2/1, concat3/1
  slice4/1 -> concat2/2
  slice13/1 -> concat2/3
  slice12/1 -> concat2/4
  cast0/1 -> concat2/5
  const0/1 -> concat2/6, concat3/6
  slice10/1 -> concat3/2
  slice15/1 -> concat3/3
  slice14/1 -> concat3/4
  cast1/1 -> concat3/5
  sync/1 -> write_counter/1, read_counter/1, block_counter/1, or0/1
  const10/1 -> read_counter/2
  write_en/1 -> write_counter/2
  block_counter/1 -> concat0/1, concat1/1
  write_counter/1 -> concat0/2, compare/1
  read_counter/1 -> concat1/2, compare1/1
  const4/1 -> compare/2
  compare/1 -> end_masking/1
  const11/1 -> compare1/2
  concat0/1 -> slice0/1, slice1/1
  slice0/1 -> cast0/1
  slice1/1 -> slice3/1
  slice3/1 -> slice4/1, slice5/1
  concat2/1 -> write_addr/1
  concat1/1 -> slice6/1, slice7/1
  slice6/1 -> cast1/1
  slice7/1 -> slice9/1
  slice9/1 -> slice10/1, slice11/1
  concat3/1 -> read_addr/1
  slice5/1 -> slice12/1, slice13/1
  slice11/1 -> slice14/1, slice15/1
  read_en/1 -> or0/2, and0/1
  or0/1 -> read_counter/4
  compare1/1 -> and0/2
  and0/1 -> read_counter/3
